simulink model "System1"  (R2021a)
settings: Solver=VariableStepAuto  StartTime=0.0  StopTime=10.0  RelTol=1e-3
values from neighbouring files (symbols this model uses):
  B = 0.1    [param.m]
  J = 100    [param.m]
  ke = 0.01    [param.m]
  kt = 0.01    [param.m]
  L = 0    [param.m]
  R = 1    [param.m]
libraries: fuzblock x1
settings Model: Creator=96171  LastModifiedBy=moham

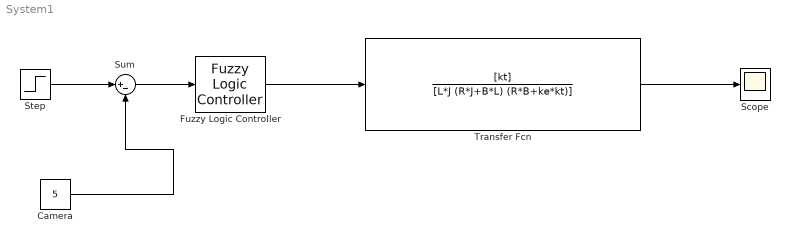
== system System1 ==
  Camera : Constant  Value=5
  Fuzzy Logic Controller : fuzblock/Fuzzy Logic  Controller  FIS=RotationController  OutputSampleNumber=101  DataType=double  FuzzifiedInputs=off  RuleFiringStrengths=off  RuleOutputs=off  AggregatedOutputs=off  SimulateUsing=Interpreted execution  OutOfRangeInputValueMessage=warning  NoRuleFiredMessage=warning  EmptyOutputFuzzySetMessage=warning
  Scope : Scope
  Step : Step  SampleTime=0
  Sum : Sum  Inputs=|+-
  Transfer Fcn : TransferFcn  Numerator=[kt]  Denominator=[L*J (R*J+B*L) (R*B+ke*kt)]
  wires:
  Transfer Fcn/1 -> Scope/1
  Fuzzy Logic Controller/1 -> Transfer Fcn/1
  Sum/1 -> Fuzzy Logic Controller/1
  Step/1 -> Sum/1
  Camera/1 -> Sum/2
